simulink model "untitled3"  (Simulink 3.00)
settings: Solver=ode45  StartTime=0.0  StopTime=10  RelTol=1e-3
settings Model: LastModifiedBy=Administrador

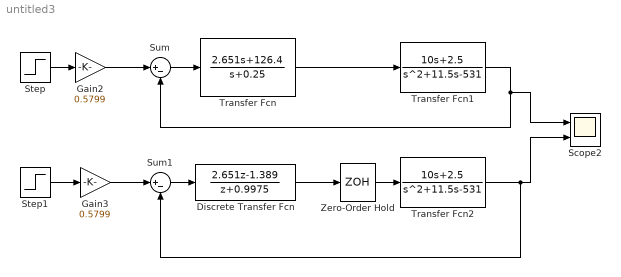
== system untitled3 ==
  Discrete Transfer Fcn : DiscreteTransferFcn  Numerator=[2.651 -1.389]  Denominator=[1 0.9975]  SampleTime=0.01
  Gain2 : Gain  Gain=0.5799  SaturateOnIntegerOverflow=on
  Gain3 : Gain  Gain=0.5799  SaturateOnIntegerOverflow=on
  Scope2 : Scope  NumInputPorts=2
      settings: TimeRange=auto  YMin=-5~-5  YMax=5~5  SaveToWorkspace=off  SaveName=ScopeData
  Step : Step  Time=0  Before=0  After=1  SampleTime=0
  Step1 : Step  Time=0  Before=0  After=1  SampleTime=0
  Sum : Sum  Inputs=|+-  SaturateOnIntegerOverflow=on
  Sum1 : Sum  Inputs=|+-  SaturateOnIntegerOverflow=on
  Transfer Fcn : TransferFcn  Numerator=[2.651 126.4]  Denominator=[1 0.25]
  Transfer Fcn1 : TransferFcn  Numerator=[10 2.5]  Denominator=[1 11.5 -531]
  Transfer Fcn2 : TransferFcn  Numerator=[10 2.5]  Denominator=[1 11.5 -531]
  Zero-Order Hold : ZeroOrderHold  SampleTime=0.25
  wires:
  Transfer Fcn/1 -> Transfer Fcn1/1
  Sum/1 -> Transfer Fcn/1
  Zero-Order Hold/1 -> Transfer Fcn2/1
  Discrete Transfer Fcn/1 -> Zero-Order Hold/1
  Sum1/1 -> Discrete Transfer Fcn/1
  Transfer Fcn1/1 -> Sum/2, Scope2/1
  Transfer Fcn2/1 -> Scope2/2, Sum1/2
  Step/1 -> Gain2/1
  Gain2/1 -> Sum/1
  Step1/1 -> Gain3/1
  Gain3/1 -> Sum1/1
